simulink model "Prescan_Carsim_0118_cs"  (R2019b)
settings: Solver=ode5  StartTime=0.0  StopTime=inf  FixedStep=1/1000  RelTol=1e-3
PreLoadFcn:
  | mbxruntime.callbacks.PreLoadFcn(bdroot);
PostLoadFcn:
  | mbxruntime.callbacks.PostLoadFcn(bdroot);
InitFcn:
  | mbxruntime.callbacks.InitFcn(bdroot);
  | Initialization_Func;
  | 
  | % load the InputBus data.
  | load osqpcecInputBus.mat;
StartFcn:
  | mbxruntime.callbacks.StartFcn(bdroot);
  | current_sys=gcs;
  | speedblock=Simulink.findBlocks(current_sys,'Name','speed_kmh_Gain');
  | h1=add_exec_event_listener(speedblock,'PostOutputs',@SpeedVisulization);
  | outblock=Simulink.findBlocks(current_sys,'Name','trajectorycurveoutput_Gain');
  | CurveTrajectoryListenerHandle=add_exec_event_listener(outblock,'PostOutputs',@TrajectoryCurve_CallBack);
  | lanedatablock=Simulink.findBlocks(current_sys,'Name','LaneData_Gain');
  | CurveLaneListenerHandle=add_exec_event_listener(lanedatablock,'PostOutputs',@CurveLane_CallBack);
StopFcn:
  | mbxruntime.callbacks.StopFcn(bdroot);
model workspace: external: MAT-File .\Prescan_Carsim_0118_cs_hws.mat (data not in the file)
values from neighbouring files (symbols this model uses):
  g = 9.8    [Initialization_Func.m]
  InitialPlanningParameter = [0,0,1,0,2,2,2,40,60]'    [Initialization_Func.m]
  Kf = 20000    [Initialization_Func.m]
  Kr = 20000    [Initialization_Func.m]
  Lr = 1.644    [Initialization_Func.m]
  M = 1275    [Initialization_Func.m]
  nG = 24    [Initialization_Func.m]
  V = 60/3.6    (= 16.6666666667)    [Initialization_Func.m]
  VehicleBaseLength = Lf+Lr    (= 2.66)    [Initialization_Func.m]
undefined symbols (not defined in the file or in its folder): AAx, AAy, AAz, AVx, AVy, AVz, Ax, Ay, Az, canChannel, DiscIntNeverNeededParam, InitialDPMPDF_Comfort, InitialDPMPDF_Efficiency, InitialDPMPDF_Safety, InitialPDF_DEM, mbxruntime, NormalisedTrajectoryIndicator_Pool, Parameter_Indicator_LookUpTable, Prescan_Carsim_1230_cs_0658e9ca1334a8be, Prescan_Carsim_1230_cs_08c5eb9a1bd7376a, Prescan_Carsim_1230_cs_6cfd759b89b9fc85, Prescan_Carsim_1230_cs_9435cc1cceb5050d, Prescan_Carsim_1230_cs_ac716d34d49f74ab, Prescan_Carsim_1230_cs_be02757d7f212dd5, Rational_Coefficient_Learning, SteeringWheel, TrajectoryIndicatorRange, Vx, Vy, Vz, WheelL0, WheelL1, WheelR0, WheelR1
libraries: canmsglib x11, dsparch4 x6, canlib x3, PreScanSimulinkLibrary x3, Solver_SF x1, autolibshared x1
(part 6 of 8)

== matlab function Prescan_Carsim_0118_cs/BMW_X5_SUV_1/DEM updating and Preference Estimation/UpdateDEM/online DPM building preference estimation accordign to feedback/MATLAB Function ==
  data: FeedBack input; Real_Trajectory_Indicator input size=[1 3]; NormalisedTrajectoryIndicator_Pool input; ExpectedNext_NormalisedTrajectoryIndicator output; ExpectedNext_QueryID output; InitialPDF_DEM input; InitialDPMPDF_Safety input size=[1 2]; InitialDPMPDF_Comfort input size=[1 2]; InitialDPMPDF_Efficiency input size=[1 2]; TrajectoryIndicatorRange input; PostPDF_DEM output; PostDPMPDF_Safety output; Rational_Coefficient_Learning input; PostDPMPDF_Comfort output; PostDPMPDF_Effociency output
function [ExpectedNext_NormalisedTrajectoryIndicator,ExpectedNext_QueryID,PostPDF_DEM,PostDPMPDF_Safety,PostDPMPDF_Comfort,PostDPMPDF_Effociency]= fcn(FeedBack,Real_Trajectory_Indicator,NormalisedTrajectoryIndicator_Pool,InitialPDF_DEM,InitialDPMPDF_Safety,InitialDPMPDF_Comfort,InitialDPMPDF_Efficiency,TrajectoryIndicatorRange,Rational_Coefficient_Learning)
% Update the PDF_DEM and PDF_DPM according to the feedback, also select the
% trajectory indicators that would be shown to the driver for the following
% evaluation (compare)
% Query: The Trajectory Indicators array Num_Indicators*1;
% InitialPDF_DEM: a data array Num_WeightDEM*4, the first column is the
% pdf,and the 2-4 column are the weight of S-C-E
% InitialPDF_DPM: a 1*3 cell array, each cell is a data array like the
% PDF_DEM.

%============ Initialization ==============
persistent PriorPDF_DEM 
if isempty(PriorPDF_DEM)
    PriorPDF_DEM=InitialPDF_DEM;
end

persistent PriorDPMPDF_Safety
if isempty(PriorDPMPDF_Safety)
    PriorDPMPDF_Safety=InitialDPMPDF_Safety;
end

persistent PriorDPMPDF_Comfort
if isempty(PriorDPMPDF_Comfort)
    PriorDPMPDF_Comfort=InitialDPMPDF_Comfort;
end

persistent PriorDPMPDF_Efficiency
if isempty(PriorDPMPDF_Efficiency)
    PriorDPMPDF_Efficiency=InitialDPMPDF_Efficiency;
end

persistent Evaluated_NormalisedTrajectoryIndicator Step
if isempty(Evaluated_NormalisedTrajectoryIndicator)
    Step=1; 
    Evaluated_NormalisedTrajectoryIndicator=zeros(size(NormalisedTrajectoryIndicator_Pool,1),1);
    Real_NormalisedTrajectory_Indicator=DriverPerceptionModel(Real_Trajectory_Indicator,0,TrajectoryIndicatorRange);
    Diff_TrajectoryInd=NormalisedTrajectoryIndicator_Pool-repmat(Real_NormalisedTrajectory_Indicator,size(NormalisedTrajectoryIndicator_Pool,1),1);
    [~,Minimum_No]=min(sum(Diff_TrajectoryInd.^2,2));
    Evaluated_NormalisedTrajectoryIndicator(Step)=Minimum_No;      
end

persistent LastPreference_TrajectoryIndicator LastPreference_NormalisedTrajectoryIndicator
if isempty(LastPreference_TrajectoryIndicator)
    LastPreference_TrajectoryIndicator=Real_Trajectory_Indicator;
    LastPreference_NormalisedTrajectoryIndicator=DriverPerceptionModel(LastPreference_TrajectoryIndicator,0,TrajectoryIndicatorRange);
end
    
persistent PDF_WeightTable ID_PDFTable
if isempty(PDF_WeightTable)
    % Construct the WeightTable and the PDF_WeightTable by combining the
    % PDF_DEM and PDF_DPM
    Num_WeightDEM=size(PriorPDF_DEM,1);
    NumIndicator_DPM=[size(PriorDPMPDF_Safety,2)-1,size(PriorDPMPDF_Comfort,2)-1,size(PriorDPMPDF_Efficiency,2)-1];% zeros means only 1 indicator
    Num_WeightDPM=[size(PriorDPMPDF_Safety,1),size(PriorDPMPDF_Comfort,1),size(PriorDPMPDF_Efficiency,1)];
    PDF_WeightTable=zeros(prod(Num_WeightDPM)*Num_WeightDEM,sum(NumIndicator_DPM)+1);
    [X1,X2,X3,X4]=ndgrid((1:Num_WeightDPM(1))',(1:Num_WeightDPM(2))',(1:Num_WeightDPM(3))',(1: Num_WeightDEM)');
    ID_PDFTable=[X1(:),X2(:),X3(:),X4(:)];
    PDF_WeightTable(:,1)=PriorDPMPDF_Safety(X1(:),1).*PriorDPMPDF_Comfort(X2(:),1).*PriorDPMPDF_Efficiency(X3(:),1).*PriorPDF_DEM(X4(:),1);
    PDF_WeightTable(:,2:end)=[(PriorDPMPDF_Safety(X1(:),2:end).*PriorPDF_DEM(X4(:),2)),(PriorDPMPDF_Comfort(X2(:),2:end).*PriorPDF_DEM(X4(:),3)),...
        (PriorDPMPDF_Efficiency(X3(:),2:end).*PriorPDF_DEM(X4(:),4))];% The last three column is the weight of S-C-E 
end


% ============= Update the PDF_DEM and PDF_DPM =====================
% feedback:1 means prefer the first one, 2 means the second one, 3 means no preference,others menas no valid feedback
if FeedBack==1 || FeedBack==2 || FeedBack==3
    Step=Step+1;    
    % Calculate the current query position
    Real_NormalizedTrajectoryIndicator=DriverPerceptionModel(Real_Trajectory_Indicator,0,TrajectoryIndicatorRange);
    Diff_TrajectoryInd=NormalisedTrajectoryIndicator_Pool-repmat(Real_NormalizedTrajectoryIndicator,size(NormalisedTrajectoryIndicator_Pool,1),1);
    [~,Minimum_No]=min(sum(Diff_TrajectoryInd.^2,2));
    Evaluated_NormalisedTrajectoryIndicator(Step)=Minimum_No;
    
    if FeedBack==1 || FeedBack==2 
        Query=Real_NormalizedTrajectoryIndicator-LastPreference_NormalisedTrajectoryIndicator;
        % When Feedback is valid,update the PDF_DEM and PDF_DPM
        Compare_Result=FeedBack-1;% prefer the latter one? 1,means the second one
        LikeHood_Feedback=LikeHood_Func(PDF_WeightTable(:,2:end),Query,Compare_Result,Rational_Coefficient_Learning);
        Post_PDFWeight=PDF_WeightTable(:,1).*LikeHood_Feedback;
        % Update the PDF_DEM and PDF_DPM
        [PostPDF_DEM,~,PostDPMPDF_Safety,PostDPMPDF_Comfort,PostDPMPDF_Effociency,~]=UpdataPDF(Post_PDFWeight,PriorPDF_DEM,PriorDPMPDF_Safety,PriorDPMPDF_Comfort,PriorDPMPDF_Efficiency,ID_PDFTable); 
        %===
        PriorPDF_DEM=PostPDF_DEM;
        PriorDPMPDF_Safety=PostDPMPDF_Safety;
        PriorDPMPDF_Comfort=PostDPMPDF_Comfort;
        PriorDPMPDF_Efficiency=PostDPMPDF_Effociency;
        if FeedBack==2          
            LastPreference_TrajectoryIndicator=Real_Trajectory_Indicator;
            LastPreference_NormalisedTrajectoryIndicator=DriverPerceptionModel(LastPreference_TrajectoryIndicator,0,TrajectoryIndicatorRange);
        end        
    else
        % Do nothing,continue the next 
    end
    
end
PostPDF_DEM=PriorPDF_DEM;
PostDPMPDF_Safety=PriorDPMPDF_Safety;
PostDPMPDF_Comfort=PriorDPMPDF_Comfort;
PostDPMPDF_Effociency=PriorDPMPDF_Efficiency;

%======= Select the Next Trajectory Used to Commare for the next loop
%=================
% 1, Calculate the expected information difference for each possible query
% This one needs further modification
Available_ID=setdiff((1:size(NormalisedTrajectoryIndicator_Pool,1)),unique(Evaluated_NormalisedTrajectoryIndicator));
Alternative_Query=NormalisedTrajectoryIndicator_Pool(Available_ID,:)-repmat(LastPreference_NormalisedTrajectoryIndicator,length(Available_ID),1);
Max_QueryID=Select_ExpectedInformationVolume(PriorPDF_DEM,PriorDPMPDF_Safety,PriorDPMPDF_Comfort,PriorDPMPDF_Efficiency,PDF_WeightTable,ID_PDFTable,Alternative_Query,Rational_Coefficient_Learning);
ExpectedNext_QueryID=Available_ID(Max_QueryID);
ExpectedNext_NormalisedTrajectoryIndicator=NormalisedTrajectoryIndicator_Pool(ExpectedNext_QueryID,:);

end


%%
% Local Functions
function likehood= LikeHood_Func(WeightSet,Query,CompareResult,Rational_Coefficient_Learning)
% calculate each query's likolihood when the result was compare(0/1)
% WeightSet: should be column vecotrs Num_Weight*Num_Indicators,
% Query: should be a data array like Num_query*Num_Indicators
% 
% likehood is a data array like Num_Weight* Num_query, 
%     beta=5;% rationality coefficient 
coder.extrinsic('error');
    likehood=1./(1+exp(Rational_Coefficient_Learning*WeightSet*Query'));
    if CompareResult ==1
        return        
    elseif CompareResult==0
        likehood=1-likehood;
    else
        error ('False compare result!\n')
    end
end

function [PostPDF_DEM,SumPDFDEM_Post,PostPDFDPM_Safety,PostPDFDPM_Comfort,PostPDFDPM_Efficiency,SumDPMPDF_Post]=UpdataPDF(Post_PDFWeight,PriorPDF_DEM,PriorDPMPDF_Safety,PriorDPMPDF_Comfort,PriorDPMPDF_Efficiency,ID_PDFTable)
% Update the PDF_DEM
PostPDF_DEM=PriorPDF_DEM;
Num_Query=size(Post_PDFWeight,2);
if not(isempty(PriorPDF_DEM))
    Num_WeightDEM_temp=size(PriorPDF_DEM,1);
    % update the DEM
    PostPDF_DEMTemp=zeros(Num_WeightDEM_temp,Num_Query);
    for DEM_i=1:Num_WeightDEM_temp
        PostPDF_DEMTemp(DEM_i,:)=sum(Post_PDFWeight(ID_PDFTable(:,4)==DEM_i,:));
    end
    [PostPDF_DEMTemp,SumPDFDEM_Post]=PDF_NormFunc(PostPDF_DEMTemp,PriorPDF_DEM(:,2:end));
end
PostPDF_DEM(:,1)=PostPDF_DEMTemp;

% update the PDF_DPM
SumDPMPDF_Post=zeros(3,Num_Query);% 3*Num_Query
Num_WeightDPM=[size(PriorDPMPDF_Safety,1),size(PriorDPMPDF_Comfort,1),size(PriorDPMPDF_Efficiency,1)];

% Update the PDFDPM_Safety
PostPDFDPM_Safety=PriorDPMPDF_Safety;
PostPDF_DPMTemp=zeros(Num_WeightDPM(1),Num_Query);
for NumWeight_i=1:Num_WeightDPM(1)
    PostPDF_DPMTemp(NumWeight_i,:)=sum(Post_PDFWeight(ID_PDFTable(:,1)==NumWeight_i,:));
end
[PostDPMPDFWeight_Temp,SumPostPDFDPM_Temp]=PDF_NormFunc(PostPDF_DPMTemp,PriorDPMPDF_Safety(:,2:end));
PostPDFDPM_Safety(:,1)=PostDPMPDFWeight_Temp;
SumDPMPDF_Post(1,:)=SumPostPDFDPM_Temp;

% Update the PDFDPM_Comfort
PostPDFDPM_Comfort=PriorDPMPDF_Comfort;
PostPDF_DPMTemp=zeros(Num_WeightDPM(2),Num_Query);
for NumWeight_i=1:Num_WeightDPM(2)
    PostPDF_DPMTemp(NumWeight_i,:)=sum(Post_PDFWeight(ID_PDFTable(:,2)==NumWeight_i,:));
end
[PostDPMPDFWeight_Temp,SumPostPDFDPM_Temp]=PDF_NormFunc(PostPDF_DPMTemp,PriorDPMPDF_Comfort(:,2:end));
PostPDFDPM_Comfort(:,1)=PostDPMPDFWeight_Temp;
SumDPMPDF_Post(2,:)=SumPostPDFDPM_Temp;

% Update the PDFDPM_Efficiency
PostPDFDPM_Efficiency=PriorDPMPDF_Efficiency;
PostPDF_DPMTemp=zeros(Num_WeightDPM(3),Num_Query);
for NumWeight_i=1:Num_WeightDPM(3)
    PostPDF_DPMTemp(NumWeight_i,:)=sum(Post_PDFWeight(ID_PDFTable(:,3)==NumWeight_i,:));
end
[PostDPMPDFWeight_Temp,SumPostPDFDPM_Temp]=PDF_NormFunc(PostPDF_DPMTemp,PriorDPMPDF_Efficiency(:,2:end));
PostPDFDPM_Efficiency(:,1)=PostDPMPDFWeight_Temp;
SumDPMPDF_Post(3,:)=SumPostPDFDPM_Temp;
end

function [post_prob,sum_prob]=PDF_NormFunc(PDF,Weight_Set)
    % prob_distrib is a array of the post probability distribution. the row
    % number is the dicrete weight number,and the column number is the query/action.
    % each column is the post prob distribution of the query.
    % this function is to calculate the total prob in the considering
    % weight range to be 1
    % pdf_func: is a function handle.
   if size(PDF,1)==1
        post_prob=1;
        sum_prob=PDF;
    else
        uniqueweight=unique(Weight_Set(:,1));
        Interval_Weight=min(diff(uniqueweight));
        Ndim_ValidWeight=size(Weight_Set,2)-1;
        % considering the truth that the valid range of the independent variable
        if Ndim_ValidWeight==1
            sum_prob=sum(PDF(1:end-1))*Interval_Weight;
        else 
            pos_temp=sum(Weight_Set(:,1:Ndim_ValidWeight),2)<=1-Interval_Weight;
            sum_prob=sum(PDF(pos_temp,:))*Interval_Weight^Ndim_ValidWeight;
        end
        post_prob=PDF./repmat(sum_prob,size(PDF,1),1);
    end        
end

function max_queryID=Select_ExpectedInformationVolume(PriorPDF_DEM,PriorDPMPDF_Safety,PriorDPMPDF_Comfort,PriorDPMPDF_Efficiency,PDF_WeightTable,ID_PDFTable,Query_Pool,learning_rate_agent)
% calculate the expected difference between the prior and post probability
% density function for each query in the Query_Pool.
% PriorPDF_DEM: initial prob distribution of the DEM(S-C-E),Num_Weight_DEM*1;
% DEM_WeightSet : date array like Ndim*Num_discrete_theta
% Query_pool:data array like Ndim*Num_query
Num_Query=size(Query_Pool,1);
DEM_WeightSet=PriorPDF_DEM(:,2:end);
Num_WeightDEM=size(PriorPDF_DEM,1);

PDF_WeightTable(:,1)=PriorDPMPDF_Safety(ID_PDFTable(:,1),1).*PriorDPMPDF_Comfort(ID_PDFTable(:,2),1).*PriorDPMPDF_Efficiency(ID_PDFTable(:,3),1).*PriorPDF_DEM(ID_PDFTable(:,4),1);
LikeHood_1_WeightByQuery=LikeHood_Func(PDF_WeightTable(:,2:end),Query_Pool,1,learning_rate_agent);
Post_PDF=repmat(PDF_WeightTable(:,1),1,Num_Query).*LikeHood_1_WeightByQuery;

% the expected information difference of DEM
PostPDF_DEM=zeros(Num_WeightDEM,Num_Query);
for DEM_i=1:Num_WeightDEM
    PostPDF_DEM(DEM_i,:)=sum(Post_PDF(ID_PDFTable(:,4)==DEM_i,:),1);
end

[Post_PDFNorm,sum_post]=PDF_NormFunc(PostPDF_DEM,DEM_WeightSet);


Prob_Difference=abs(repmat(PriorPDF_DEM(:,1),1,Num_Query)-Post_PDFNorm);
[~,Sum_Prob_Difference]=PDF_NormFunc(Prob_Difference,DEM_WeightSet);
Expected_Information=Sum_Prob_Difference.*sum_post;
[~,max_queryID]=max(Expected_Information);
end

function TrajectoryIndicator_Perceived=DriverPerceptionModel(TrajectoryIndicator,Flag,TrajectoryIndicatorRange)
% Flag: 0 means to transform the real trajectory indicator into Normalized
% Trajectory Indicators, vice versa, 1 means transform the normalized into
% real trajectory indicators

% RightLateralOffset,LateralAcceleration,Time
% Minimum_TrajectoryIndicator=[0,0.4,14];
% Maximum_TrajectoryIndicator=[0.5,3.4,18];
Minimum_TrajectoryIndicator=TrajectoryIndicatorRange(1,:);
Maximum_TrajectoryIndicator=TrajectoryIndicatorRange(2,:);

if Flag==1
    Normalized_TrajectoryIndicator=TrajectoryIndicator;
    TrajectoryIndicator_Perceived=Minimum_TrajectoryIndicator+(Maximum_TrajectoryIndicator-Minimum_TrajectoryIndicator).*Normalized_TrajectoryIndicator;
    % This is special for the LateralOffset_Right
    TrajectoryIndicator_Perceived(1)=-1*TrajectoryIndicator_Perceived(1);
elseif Flag==0
    %==== These are refered to the DriverPerceptionBase.m
    % JND-just noticeable difference
    %Can You Feel The Difference? The Just Noticeable Difference of
    %Longitudinal Acceleration, http://sage.cnpereading.com/paragraph/article/?doi=10.1177/1541931213571271
    JND_Acceleration=0.1;
    % Lateral Offset, Assume Left and Right be tha same,and to be 0.1m;
    JND_LateralOffset=0.1;%
    % Time, Or May be the Average Time would be More Significant
    JND_Time=2;
    
    GridIndicator=zeros(3,size(Minimum_TrajectoryIndicator,2));
    GridIndicator(1,:)=(Minimum_TrajectoryIndicator+eps)./[JND_LateralOffset,JND_Acceleration,JND_Time];
    GridIndicator(2,:)=(Maximum_TrajectoryIndicator+eps)./[JND_LateralOffset,JND_Acceleration,JND_Time];
    GridIndicator(3,:)=(abs(TrajectoryIndicator)+eps)./[JND_LateralOffset,JND_Acceleration,JND_Time];
    
    TrajectoryIndicator_Perceived=(GridIndicator(3,:)-GridIndicator(1,:))./(GridIndicator(2,:)-GridIndicator(1,:));
    TrajectoryIndicator_Perceived(TrajectoryIndicator_Perceived<0)=0;
    TrajectoryIndicator_Perceived(TrajectoryIndicator_Perceived>1)=1;
end
end

== matlab function Prescan_Carsim_0118_cs/BMW_X5_SUV_1/trajectory planning/A substitution for the above trajectory planning subsystem/Trajectory Planning When Not Curve ==
  data: RoadLane_Plan input size=[1000 4]; Path_Plan output size=[1000 2]; Speed_Planned_kmh output size=[1000 1]; MaxSpeed input; PlanPathDataLength_Straight output size=1
function [Path_Plan,Speed_Planned_kmh,PlanPathDataLength_Straight]= fcn(RoadLane_Plan,MaxSpeed)

%Road Lane
LeftLane_Plan=RoadLane_Plan(:,1:2);
RightLane_Plan=RoadLane_Plan(:,3:4);
Num_LanePlan=size(RightLane_Plan,1);
Path_PlanTemp=zeros(1000,2);

X_LeftToRight=RightLane_Plan(:,1)-LeftLane_Plan(:,1);%const 2
Y_LeftToRight=RightLane_Plan(:,2)-LeftLane_Plan(:,2);

alpha=0.5*ones(Num_LanePlan,1); % Lane centering
Path_PlanTemp(1:Num_LanePlan,1) = LeftLane_Plan(:,1) + X_LeftToRight.* alpha;
Path_PlanTemp(1:Num_LanePlan,2)= LeftLane_Plan(:,2) + Y_LeftToRight.* alpha;
% Path_Plan=Path_PlanTemp(1:Num_LanePlan,:);
Path_Plan=Path_PlanTemp;
PlanPathDataLength_Straight=Num_LanePlan;
% Speed_Planned_kmh=Constant_Speed*ones(Num_LanePlan,1);
Speed_Planned_kmh=MaxSpeed*ones(1000,1);
%Trajectory=[Path_Plan,Speed_Planned_kmh];

% smooth or interplate the trajecotry 

end

== matlab function Prescan_Carsim_0118_cs/BMW_X5_SUV_1/trajectory planning/Specific Curve Trajectory Planning/Convert Curve Path To Local (under vehicle) ==
  data: PathPlan_Global input size=[1000 2]; VehicleState_Global input; PathPlan_Local output size=[1000 2]
function PathPlan_Local =fcn(PathPlan_Global,VehicleState_Global)
% Convert the global path to local(different with the local under beginning
%  position.
X_TargetPath=PathPlan_Global(:,1);
Y_TargetPath=PathPlan_Global(:,2);
HeadingAngle_rad=VehicleState_Global(3);
PathPlan_Local =([X_TargetPath - VehicleState_Global(1),Y_TargetPath-VehicleState_Global(2)])*[cos(HeadingAngle_rad) sin(HeadingAngle_rad); -sin(HeadingAngle_rad) cos(HeadingAngle_rad)]';  % 将原始参考路径旋转平移至车辆坐标系下
end

== matlab function Prescan_Carsim_0118_cs/BMW_X5_SUV_1/trajectory planning/Subsystem/Determination of Curve Road No/Determine Curve No According the vehicle position ==
  data: VehicleState_Global input; Curve_No output
function Curve_No = fcn(VehicleState_Global)
X_Global=VehicleState_Global(1);
Y_Global=VehicleState_Global(2);
% These coordinates was from the scenery in pex GUI
if X_Global>=20 && Y_Global>=-182.7
    %Y_Global>=150 && Y_Global<=300.6
    % This is not very accurate
    Curve_No=1;
elseif X_Global>=20 && Y_Global<=-272.7
    %Y_Global>=400.6 && Y_Global<=554.247
    Curve_No=2;
elseif X_Global<=-70 && Y_Global<=-272.7
    Curve_No=3;
elseif X_Global<=-70 && Y_Global>=-182.7
    Curve_No=4;    
else
    Curve_No=0;
end

== matlab function Prescan_Carsim_0118_cs/BMW_X5_SUV_1/trajectory tracking Information/Preview Information Calculation 2 ==
  data: TargetPath_Local input size=[1000 2]; Offset_Preview output; HeadError_rad output; Curvature_Vehicle output; TargetSpeed_Plan input size=[1000 1]; TrackingError output; PreviewDistance output; TargetSpeed_Current output
function [Offset_Preview,HeadError_rad,Curvature_Vehicle,TrackingError,PreviewDistance,TargetSpeed_Current] = fcn(TargetPath_Local,TargetSpeed_Plan)
% calculate the preview information used in the SMC controller

Path_UnderVehicleCoordinates=TargetPath_Local;
% Target speed for current vehicle position
% Pick up the speed points close to the vehicle, within range(-15,15)
Speed_CloseToVehicle= TargetSpeed_Plan(Path_UnderVehicleCoordinates(:,1)<=15 ...
    & Path_UnderVehicleCoordinates(:,1)>=-15,:);
ID_CloseToVehicle= Path_UnderVehicleCoordinates(Path_UnderVehicleCoordinates(:,1)<=15 ...
    & Path_UnderVehicleCoordinates(:,1)>=-15,:);
% % spline
TargetSpeed_Current = spline(ID_CloseToVehicle(:,1), Speed_CloseToVehicle, 0);% current speed
PreviewDistance=0.072*TargetSpeed_Current+5;% used to calculate the preview error

%Pick up the path points close to the preview point
Path_CloseToPreview= Path_UnderVehicleCoordinates(Path_UnderVehicleCoordinates(:,1)<= 2*PreviewDistance & Path_UnderVehicleCoordinates(:,1)>=0,:);
%spline
Interval_spline = 0.01;
Xeq = (0 : Interval_spline : Path_CloseToPreview(end,1))';
Yeq = spline(Path_CloseToPreview(:,1), Path_CloseToPreview(:,2), Xeq);
PathCloseToPreview_spline=[Xeq,Yeq];
%Calculate the lateral offset of the preview point，
%Positive if the preview point is on the left of the target path,vice versa
Preview_Point=[PreviewDistance,0];
[Offset_Preview,~,~]=DistanceCurvature_Calculate(PathCloseToPreview_spline,Preview_Point,0,0);


%Calculate the curvature of the target path that close to the vehicle,
% Positive if the target path curve is left curve, vice versa
%Pick up the path points close to the vehicle
Path_CloseToVehicle= Path_UnderVehicleCoordinates(Path_UnderVehicleCoordinates(:,1)<=2*PreviewDistance ...
    & Path_UnderVehicleCoordinates(:,1)>=-2*PreviewDistance,:);
%spline
Xeq = (-2*PreviewDistance : Interval_spline : Path_CloseToVehicle(end,1))';
Yeq = spline(Path_CloseToVehicle(:,1), Path_CloseToVehicle(:,2), Xeq);
PathCloseToVehicle_spline=[Xeq,Yeq];
[TrackingError,Curvature_Vehicle,HeadError_rad]=DistanceCurvature_Calculate(PathCloseToVehicle_spline,[0,0],1,1);

% Visulization
% Plot_Preview_Local(TargetPath_Local,Distance_Preview)
end

%%
%local functions
function [DistanceToPoint,Curvature,HeadError]=DistanceCurvature_Calculate(Path,Target_Point,Curvature_Cal,HeadError_Cal)
% #codegen
coder.extrinsic('warning');
[~, Id_min]=min((Target_Point(1)-Path(:,1)).^2+(Target_Point(2)-Path(:,2)).^2);
if (Id_min < size(Path,1)-10)
    vec_Path = [Path(Id_min+10,:),0]-[Path(Id_min,:),0];
    vec_TargetToPath = [Target_Point,0]-[Path(Id_min,:),0];
else
    vec_Path = [Path(Id_min,:),0]-[Path(Id_min-10,:),0];
    vec_TargetToPath = [Target_Point,0]-[Path(Id_min-10,:),0];
end
Cross_VecPretoPath_VecPath=cross(vec_Path,vec_TargetToPath);
DistanceToPoint=Cross_VecPretoPath_VecPath(:,3)./sqrt(sum(vec_Path.*vec_Path));
% DistanceToPoint=sqrt(DisSquare_PreToPath);
Sin_Angle=abs(DistanceToPoint)/sqrt(sum(vec_TargetToPath.*vec_TargetToPath));
if Sin_Angle<sin(deg2rad(85))
    warning('The calcuated lateral distance of preview point to path is not very accurate!');
end

HeadError=0;
if HeadError_Cal==1
   Vec_Vehicle=[1,0,0];
%    if (Id_min < size(Path,1))
%       vec_Path2=[Path(Id_min+1,:),0]-[Path(Id_min,:),0];
%    else
%       vec_Path2 = [Path(Id_min,:),0]-[Path(Id_min-1,:),0];
%    end
   Cross_VehicleToPath=cross(vec_Path,Vec_Vehicle);
   Sin_Angle=Cross_VehicleToPath(3)/sqrt(sum(vec_Path.*vec_Path));
   HeadError=asin(Sin_Angle);   
end

Curvature=0;
if Curvature_Cal==1
    Radius_ChooseDataForCur=300;% about 3m for interval 0.01.
    if Id_min<=size(Path,1)-Radius_ChooseDataForCur && Id_min>=Radius_ChooseDataForCur
        Id_Lower=Id_min-Radius_ChooseDataForCur+1;
        Id_Upper=Id_min+Radius_ChooseDataForCur;
    elseif Id_min>size(Path,1)-Radius_ChooseDataForCur
        Id_Upper=size(Path,1);
        Id_Lower=max(size(Path,1)-2*Radius_ChooseDataForCur,1);        
    elseif Id_min<Radius_ChooseDataForCur
        Id_Lower=1;
        Id_Upper=min(2*Radius_ChooseDataForCur,size(Path,1));
    else
        warning('The curvature calculation is something wrong!');
        Curvature=0;
        return
    end
    %{
    % Method 1
    Path_cur=Path(Id_Lower:Id_Upper,:);
    A=[Path_cur,ones(size(Path_cur,1),1)];
    if rank(A) ~= size(A,2)
        Curvature= 0;
    else
        B=-1*sum(Path_cur.*Path_cur,2);
        coef=A\B;%圆一般方程式的的系数DEF
        Curvature=2/sqrt(coef(1)^2+coef(2)^2-4*coef(3));
        if Curvature<1/1000
            Curvature=0;
        end
    end
    %}
    % Method 2 another method with 3 points, but maybe unstable
    vec1 = [Path(Id_min,:)-Path(Id_Lower,:),0];
    vec2 = [Path(Id_Upper,:)-Path(Id_min,:),0];
    z1 =Path(Id_min,:)*Path(Id_min,:)'-Path(Id_Lower,:)*Path(Id_Lower,:)';
    z2 =Path(Id_Upper,:)*Path(Id_Upper,:)'-Path(Id_Lower,:)*Path(Id_Lower,:)';
    z3 =Path(Id_Upper,:)*Path(Id_Upper,:)'-Path(Id_min,:)*Path(Id_min,:)'; 
    direction  = cross(vec1,vec2);
    sin_theta=abs(direction(3))/(sqrt(vec1*vec1')*sqrt(vec2*vec2'));
    curvature_estimate=asin(sin_theta)/(sqrt(vec2*vec2'));% the theta/length
    if curvature_estimate>1/1000  
        % the curvatrue_estimate is larger than 1/1000(Radius is smaller than 1000),the old is the direction(3) is
        % larger than 1e-9;
        A = [Path(Id_min,:)-Path(Id_Lower,:); Path(Id_Upper,:)-Path(Id_Lower,:); Path(Id_Upper,:)-Path(Id_min,:)];
        B = 0.5*[z1;  z2;  z3];
        P0 = (A'*A)\A'*B;
        R1 =sqrt((P0'-Path(Id_Lower,:))*(P0'-Path(Id_Lower,:))');
        R2 =sqrt((P0'-Path(Id_min,:))*(P0'-Path(Id_min,:))');
        R3 =sqrt((P0'-Path(Id_Upper,:))*(P0'-Path(Id_Upper,:))');
        R = (R1 + R2 + R3)/3;
        Curvature = 1/R*sign(direction(3));
    else
        Curvature = 0;
    end
    %}
end
end

== matlab function Prescan_Carsim_0118_cs/BMW_X5_SUV_1/Tracking Control & vehicle dynamics/Lane Keeping Assistance/Path Tracking - SMC controller ==
  data: c1 input; c2 input; delta input; kapa input; PreviewError input; PreviewError_dot input; HeadingError input; HeadingError_dot input; Curvature input; SteerAngle output; PreviewDistance input; v input
function SteerAngle = fcn( c1, c2, delta, kapa, PreviewError, PreviewError_dot, HeadingError, HeadingError_dot, Curvature,PreviewDistance,v)
% 滑膜控制参数定义
%先定义车辆本身的参数
g=9.8;%重力加速度m/s^2
M=1396; %车辆的质量kg
I=2204; %车辆的横摆转动惯量kg·m2
Kf=50192; %前轮的侧偏刚度Nm/rad
Kr=50192; %后轮的侧偏刚度Nm/rad
Lf=1.01; %车辆质心到前轴的距离m
Lr=1.59; %车辆质心到后轴的距离m
%待调参数： 预瞄时长t_pre, 滑膜面参数 c1, c2, 趋近率参数delta, kapa
%输入参数； 预瞄偏差ep,  参考航向角phi_d, 本车航向角 phi, 道路曲率 qulv  航向角偏差影响系数 phir_k0 phir_k1
phir_k0 = 0.85;
phir_k1 = 0.85;
L = PreviewDistance; %车辆预瞄距离设定
smc_a12 = -(1+(Lf*Kf-Lr*Kr)/(M*v^2));
smc_a34 = (Kf+Kr)/M+L*(Kf*Lf-Kr*Lr)/I;
smc_a35 = L*(Kf+Kr)/(M*v)-(Kf*Lf-Kr*Lr)/(M*v)+L^2*(Kf*Lf-Kr*Lr)/(I*v)-L*(Kf*Lf^2+Kr*Lr^2)/(I*v);
smc_a36 = (Kf+Kr)/(M*v)+L*(Kf*Lf-Kr*Lr)/(I*v);
smc_b32 = (L*Kf*Lf)/I+Kf/M;
smc_d32 = -(v+(Kf*Lf-Kr*Lr)/(M*v)-L*smc_a12);
ep_cum = 0;
s1 = PreviewError_dot + c1 * PreviewError + c2 * ep_cum;
f1 = smc_a34 * HeadingError*phir_k0 + smc_a35 * HeadingError_dot*phir_k1 + c2 * PreviewError + (smc_a36+c1)*PreviewError_dot;
t1 = (1-exp(-10*s1))./(1+exp(-10*s1));
smc_ur = -1/smc_b32*(delta*t1 + kapa*s1 + f1 + smc_d32*v*Curvature);
k3 = smc_a34/smc_b32;
smc_uf = (M*v^2*Curvature)/(2*(Lf+Lr))*(Lr/Kf-Lf/Kr+Lf/Kr*k3)+Curvature*((Lf+Lr)-Lr*k3);
smc_u = smc_uf*0.03*(0) + smc_ur;
SteerAngle = smc_u;

== matlab function Prescan_Carsim_0118_cs/BMW_X5_SUV_1/trajectory planning/A substitution for the above trajectory planning subsystem/Convert Curve Path To Local (under vehicle) ==
  data: PathPlan_Global input size=[1000 2]; VehicleState_CurvePlanningBegining input size=[1 3]; VehicleState_Global input; PathPlan_Local output size=[1000 2]
function PathPlan_Local =fcn(PathPlan_Global,VehicleState_CurvePlanningBegining,VehicleState_Global)
% #codegen
% Convert the local path to global path
HeadingAngle_Beginning_rad=deg2rad(VehicleState_CurvePlanningBegining(3));
Rotation_Beginning=[cos(HeadingAngle_Beginning_rad),-sin(HeadingAngle_Beginning_rad); sin(HeadingAngle_Beginning_rad),cos(HeadingAngle_Beginning_rad)];
PathPlan_Beginning_temp=PathPlan_Global(:,1:2)*Rotation_Beginning';
PathPlan_Beginning=[PathPlan_Beginning_temp(:,1)+VehicleState_CurvePlanningBegining(1),...
    PathPlan_Beginning_temp(:,2)+VehicleState_CurvePlanningBegining(2)];

% Convert the global path to local(different with the local under beginning
%  position.
X_TargetPath=PathPlan_Beginning(:,1);
Y_TargetPath=PathPlan_Beginning(:,2);
HeadingAngle_rad=deg2rad(VehicleState_Global(3));
PathPlan_Local =([X_TargetPath - VehicleState_Global(1),Y_TargetPath-VehicleState_Global(2)])*[cos(HeadingAngle_rad) sin(HeadingAngle_rad); -sin(HeadingAngle_rad) cos(HeadingAngle_rad)]';  % 将原始参考路径旋转平移至车辆坐标系下
end

== matlab function Prescan_Carsim_0118_cs/BMW_X5_SUV_1/trajectory planning/A substitution for the above trajectory planning subsystem/MATLAB Function ==
  data: PathPlan_FixedSize input; TargetPath_VariableSize output size=[1000 2]; PlanSpeed_FixedSize input; TargetSpeed_VariableSize output size=[1000 1]; DataLength_Plan input
function [TargetPath_VariableSize,TargetSpeed_VariableSize]  = fcn(PathPlan_FixedSize,PlanSpeed_FixedSize,DataLength_Plan)
TargetPath_VariableSize=PathPlan_FixedSize(1:DataLength_Plan,:);
TargetSpeed_VariableSize = PlanSpeed_FixedSize(1:DataLength_Plan,:);
end

== matlab function Prescan_Carsim_0118_cs/BMW_X5_SUV_1/DriverFeedBack/driver evaluation model/Simulated Driver ==
  data: TrajectoryIndicator input size=[1 3]; Preference_DEM input; Compare_Result output; FeedBack_Count output; PreferenceDPM_Safety input; PreferenceDPM_Comfort input; PreferenceDPM_Efficiency input; Rational_coefficient input; Driver_Type input; mis_answered_ind output
function [Compare_Result,FeedBack_Count,mis_answered_ind]=Driver_Compare(TrajectoryIndicator,Preference_DEM,PreferenceDPM_Safety,PreferenceDPM_Comfort,PreferenceDPM_Efficiency,Rational_coefficient,Driver_Type)
%#codegen
% preference should be a column vector Ndim*1;
% query should be a data array Ndim*Num_query
% varargin- 'driver type', the list value include{'complete_rational','probability_rational','bound_rational'}
%  'bound_rational': when the probability of prefered is larger than a
%  upper_bound, the answer is 1; or when the probability of prefered is
%  less than a lower bound, the answer is 0; else the probability within
%  [lower_bound, upper_bound], the driver answers according to the
%  probability.
% Preference_DEM:3*1
coder.extrinsic('error');

persistent FeedBack_trigger
if isempty(FeedBack_trigger)
    FeedBack_trigger=0;
end

persistent LastPreference_TrajectoryIndicator_Driver
if isempty(LastPreference_TrajectoryIndicator_Driver)
    LastPreference_TrajectoryIndicator_Driver=TrajectoryIndicator;
end

persistent InitialFlag
if isempty(InitialFlag)
    InitialFlag=1;
end

mis_answered_ind=0;
if InitialFlag==1
    Compare_Result=-1;
    InitialFlag=0;
else    
    Query=TrajectoryIndicator-LastPreference_TrajectoryIndicator_Driver;
    Num_query=size(Query,1);
    Compare_Result=zeros(Num_query,1);
    Preference=[Preference_DEM(1)*PreferenceDPM_Safety(1,:),Preference_DEM(2)*PreferenceDPM_Comfort(1,:),Preference_DEM(3)*PreferenceDPM_Efficiency(1,:)];
    prob_1=LikeHood_Func(Preference,Query,1,Rational_coefficient);    
    if Driver_Type==1
        %"complete_rational"
        Compare_Result(prob_1>0.5)=1;
    elseif Driver_Type==2
        %"probability_rational"
        r1=rand(1,Num_query);
        Compare_Result(prob_1>r1)=1;
        False_negative=prob_1>0.5 & Compare_Result==0;
        False_positive=prob_1<0.5 & Compare_Result==1;
        mis_answered_ind=double(False_negative | False_positive);
    else 
        % "bound_rational"
        upper_bound=0.6;
        lower_bound=0.4;
        Compare_Result(prob_1>upper_bound)=1;
        prob_ind=prob_1>lower_bound & prob_1<= upper_bound;
        Compare_Result(prob_ind)=2;
        False_negative=prob_1>0.5 & Compare_Result==0;
        False_positive=prob_1<0.5 & Compare_Result==1;
        mis_answered_ind=double(False_negative | False_positive);         
    end
    if isequal(FeedBack_trigger,0)
        FeedBack_trigger=1;
    else
        FeedBack_trigger=0;
    end
end

FeedBack_Count=FeedBack_trigger;
Compare_Result=Compare_Result+1;
if Compare_Result==2
    LastPreference_TrajectoryIndicator_Driver=TrajectoryIndicator;
end
end

== matlab function Prescan_Carsim_0118_cs/BMW_X5_SUV_1/trajectory planning/Out of Specific Curve Planning/Trajectory Planning When Not Curve ==
  data: RoadLane_Plan input size=[1000 4]; Path_Plan output size=[1000 2]; Speed_Planned_kmh output size=[1000 1]; MaxSpeed input; PlanPathDataLength_Straight output size=1
function [Path_Plan,Speed_Planned_kmh,PlanPathDataLength_Straight]= fcn(RoadLane_Plan,MaxSpeed)

%Road Lane
LeftLane_Plan=RoadLane_Plan(:,1:2);
RightLane_Plan=RoadLane_Plan(:,3:4);
Num_LanePlan=size(RightLane_Plan,1);
Path_PlanTemp=zeros(1000,2);

X_LeftToRight=RightLane_Plan(:,1)-LeftLane_Plan(:,1);%const 2
Y_LeftToRight=RightLane_Plan(:,2)-LeftLane_Plan(:,2);

alpha=0.5*ones(Num_LanePlan,1); % Lane centering
Path_PlanTemp(1:Num_LanePlan,1) = LeftLane_Plan(:,1) + X_LeftToRight.* alpha;
Path_PlanTemp(1:Num_LanePlan,2)= LeftLane_Plan(:,2) + Y_LeftToRight.* alpha;
% Path_Plan=Path_PlanTemp(1:Num_LanePlan,:);
Path_Plan=Path_PlanTemp;
PlanPathDataLength_Straight=Num_LanePlan;
% Speed_Planned_kmh=Constant_Speed*ones(Num_LanePlan,1);
Speed_Planned_kmh=MaxSpeed*ones(1000,1);
%Trajectory=[Path_Plan,Speed_Planned_kmh];

% smooth or interplate the trajecotry 

end

== matlab function Prescan_Carsim_0118_cs/BMW_X5_SUV_1/DEM updating and Preference Estimation/UpdateDEM/Trajectory Planning Parameter Management1/Determine planning parameter according to the expected TrajectoryIndicators_LookUpTable ==
  data: IntialTrajectoryPlanningParameter input; PlanningParameter output; unused input; ExpectedNext_QueryID input; Parameter_IndicatorLookUpTable input
function PlanningParameter = fcn(IntialTrajectoryPlanningParameter,~,ExpectedNext_QueryID,Parameter_IndicatorLookUpTable)

persistent Parameter_Indicator_LookUpTable
if isempty(Parameter_Indicator_LookUpTable)
    Parameter_Indicator_LookUpTable=Parameter_IndicatorLookUpTable;
end
% if it is the first tiem
persistent Flag
if isempty(Flag)
    Flag=0;
end

persistent Intial_PlanningParameter
if isempty(Intial_PlanningParameter)
    Intial_PlanningParameter=IntialTrajectoryPlanningParameter;
end

if Flag==0
    PlanningParameter=Intial_PlanningParameter;
else
    PlanningParameter=Parameter_Indicator_LookUpTable(ExpectedNext_QueryID,1:9)';
end
Flag=1;
end

== matlab function Prescan_Carsim_0118_cs/BMW_X5_SUV_1/DEM updating and Preference Estimation/UpdateDEM/Online DEM updating/UPdate DEM ==
  data: FeedBack input; Query input size=[1 3]; PriorPDF_DEM input; PriorDPMPDF_Safety input size=[1 2]; PriorDPMPDF_Comfort input size=[1 2]; PriorDPMPDF_Efficiency input size=[1 2]; PostPDF_DEM output; PostDPMPDF_Safety output; Rational_Coefficient_Learning input; PostDPMPDF_Comfort output; PostDPMPDF_Effociency output
function [PostPDF_DEM,PostDPMPDF_Safety,PostDPMPDF_Comfort,PostDPMPDF_Effociency]= fcn(FeedBack,Query,PriorPDF_DEM,PriorDPMPDF_Safety,PriorDPMPDF_Comfort,PriorDPMPDF_Efficiency,Rational_Coefficient_Learning)
% Update the PDF_DEM and PDF_DPM according to the feedback, also select the
% trajectory indicators that would be shown to the driver for the following
% evaluation (compare)
% Query: The Trajectory Indicators array Num_Indicators*1;
% InitialPDF_DEM: a data array Num_WeightDEM*4, the first column is the
% pdf,and the 2-4 column are the weight of S-C-E
% InitialPDF_DPM: a 1*3 cell array, each cell is a data array like the
% PDF_DEM.

%============ Initialization ==============  

persistent Prior_DEM 
if isempty(Prior_DEM)
    Prior_DEM=PriorPDF_DEM;
end

persistent PriorDPM_Safety
if isempty(PriorDPM_Safety)
    PriorDPM_Safety=PriorDPMPDF_Safety;
end

persistent PriorDPM_Comfort
if isempty(PriorDPM_Comfort)
    PriorDPM_Comfort=PriorDPMPDF_Comfort;
end

persistent PriorDPM_Efficiency
if isempty(PriorDPM_Efficiency)
    PriorDPM_Efficiency=PriorDPMPDF_Efficiency;
end

persistent PDF_WeightTable ID_PDFTable
if isempty(PDF_WeightTable)
    % Construct the WeightTable and the PDF_WeightTable by combining the
    % PDF_DEM and PDF_DPM
    Num_WeightDEM=size(PriorPDF_DEM,1);
    NumIndicator_DPM=[size(PriorDPMPDF_Safety,2)-1,size(PriorDPMPDF_Comfort,2)-1,size(PriorDPMPDF_Efficiency,2)-1];% zeros means only 1 indicator
    Num_WeightDPM=[size(PriorDPMPDF_Safety,1),size(PriorDPMPDF_Comfort,1),size(PriorDPMPDF_Efficiency,1)];
    PDF_WeightTable=zeros(prod(Num_WeightDPM)*Num_WeightDEM,sum(NumIndicator_DPM)+1);
    [X1,X2,X3,X4]=ndgrid((1:Num_WeightDPM(1))',(1:Num_WeightDPM(2))',(1:Num_WeightDPM(3))',(1: Num_WeightDEM)');
    ID_PDFTable=[X1(:),X2(:),X3(:),X4(:)];
%   PDF_WeightTable(:,1)=PriorDPMPDF_Safety(X1(:),1).*PriorDPMPDF_Comfort(X2(:),1).*PriorDPMPDF_Efficiency(X3(:),1).*PriorPDF_DEM(X4(:),1);
    PDF_WeightTable(:,2:end)=[(PriorDPMPDF_Safety(X1(:),2:end).*PriorPDF_DEM(X4(:),2)),(PriorDPMPDF_Comfort(X2(:),2:end).*PriorPDF_DEM(X4(:),3)),...
        (PriorDPMPDF_Efficiency(X3(:),2:end).*PriorPDF_DEM(X4(:),4))];% The last three column is the weight of S-C-E 
end
PDF_WeightTable(:,1)=PriorDPMPDF_Safety(ID_PDFTable(:,1),1).*PriorDPMPDF_Comfort(ID_PDFTable(:,2),1).*PriorDPMPDF_Efficiency(ID_PDFTable(:,3),1).*PriorPDF_DEM(ID_PDFTable(:,4),1);

% ============= Update the PDF_DEM and PDF_DPM =====================
% feedback:1 means prefer the first one, 2 means the second one, 3 means no preference,others menas no valid feedback    
if FeedBack==1 || FeedBack==2 
    % When Feedback is valid,update the PDF_DEM and PDF_DPM
    Compare_Result=FeedBack-1;% prefer the latter one? 1,means the second one
    LikeHood_Feedback=LikeHood_Func(PDF_WeightTable(:,2:end),Query,Compare_Result,Rational_Coefficient_Learning);
    Post_PDFWeight=PDF_WeightTable(:,1).*LikeHood_Feedback;
    % Update the PDF_DEM and PDF_DPM
    [PostPDF_DEMtemp,~,PostDPMPDF_Safetytemp,PostDPMPDF_Comforttemp,PostDPMPDF_Effociencytemp,~]=UpdataPDF(Post_PDFWeight,PriorPDF_DEM,PriorDPMPDF_Safety,PriorDPMPDF_Comfort,PriorDPMPDF_Efficiency,ID_PDFTable); 
    Prior_DEM=PostPDF_DEMtemp;
    PriorDPM_Safety=PostDPMPDF_Safetytemp;
    PriorDPM_Comfort=PostDPMPDF_Comforttemp;
    PriorDPM_Efficiency=PostDPMPDF_Effociencytemp;
else
    % if no preference,(the two have no obvious difference)==============
    % Do nothing,continue the next 
end    

PostPDF_DEM=Prior_DEM;
PostDPMPDF_Safety=PriorDPM_Safety;
PostDPMPDF_Comfort=PriorDPM_Comfort;
PostDPMPDF_Effociency=PriorDPM_Efficiency;

end


%%
% Local Functions
function likehood= LikeHood_Func(WeightSet,Query,CompareResult,Rational_Coefficient_Learning)
% calculate each query's likolihood when the result was compare(0/1)
% WeightSet: should be column vecotrs Num_Weight*Num_Indicators,
% Query: should be a data array like Num_query*Num_Indicators
% 
% likehood is a data array like Num_Weight* Num_query, 
%     beta=5;% rationality coefficient 
coder.extrinsic('error');
    likehood=1./(1+exp(Rational_Coefficient_Learning*WeightSet*Query'));
    if CompareResult ==1
        return        
    elseif CompareResult==0
        likehood=1-likehood;
    else
        error ('False compare result!\n')
    end
end

function [PostPDF_DEM,SumPDFDEM_Post,PostPDFDPM_Safety,PostPDFDPM_Comfort,PostPDFDPM_Efficiency,SumDPMPDF_Post]=UpdataPDF(Post_PDFWeight,PriorPDF_DEM,PriorDPMPDF_Safety,PriorDPMPDF_Comfort,PriorDPMPDF_Efficiency,ID_PDFTable)
% Update the PDF_DEM
PostPDF_DEM=PriorPDF_DEM;
Num_Query=size(Post_PDFWeight,2);
if not(isempty(PriorPDF_DEM))
    Num_WeightDEM_temp=size(PriorPDF_DEM,1);
    % update the DEM
    PostPDF_DEMTemp=zeros(Num_WeightDEM_temp,Num_Query);
    for DEM_i=1:Num_WeightDEM_temp
        PostPDF_DEMTemp(DEM_i,:)=sum(Post_PDFWeight(ID_PDFTable(:,4)==DEM_i,:));
    end
    [PostPDF_DEMTemp,SumPDFDEM_Post]=PDF_NormFunc(PostPDF_DEMTemp,PriorPDF_DEM(:,2:end));
end
PostPDF_DEM(:,1)=PostPDF_DEMTemp;

% update the PDF_DPM
SumDPMPDF_Post=zeros(3,Num_Query);% 3*Num_Query
Num_WeightDPM=[size(PriorDPMPDF_Safety,1),size(PriorDPMPDF_Comfort,1),size(PriorDPMPDF_Efficiency,1)];

% Update the PDFDPM_Safety
PostPDFDPM_Safety=PriorDPMPDF_Safety;
PostPDF_DPMTemp=zeros(Num_WeightDPM(1),Num_Query);
for NumWeight_i=1:Num_WeightDPM(1)
    PostPDF_DPMTemp(NumWeight_i,:)=sum(Post_PDFWeight(ID_PDFTable(:,1)==NumWeight_i,:));
end
[PostDPMPDFWeight_Temp,SumPostPDFDPM_Temp]=PDF_NormFunc(PostPDF_DPMTemp,PriorDPMPDF_Safety(:,2:end));
PostPDFDPM_Safety(:,1)=PostDPMPDFWeight_Temp;
SumDPMPDF_Post(1,:)=SumPostPDFDPM_Temp;

% Update the PDFDPM_Comfort
PostPDFDPM_Comfort=PriorDPMPDF_Comfort;
PostPDF_DPMTemp=zeros(Num_WeightDPM(2),Num_Query);
for NumWeight_i=1:Num_WeightDPM(2)
    PostPDF_DPMTemp(NumWeight_i,:)=sum(Post_PDFWeight(ID_PDFTable(:,2)==NumWeight_i,:));
end
[PostDPMPDFWeight_Temp,SumPostPDFDPM_Temp]=PDF_NormFunc(PostPDF_DPMTemp,PriorDPMPDF_Comfort(:,2:end));
PostPDFDPM_Comfort(:,1)=PostDPMPDFWeight_Temp;
SumDPMPDF_Post(2,:)=SumPostPDFDPM_Temp;

% Update the PDFDPM_Efficiency
PostPDFDPM_Efficiency=PriorDPMPDF_Efficiency;
PostPDF_DPMTemp=zeros(Num_WeightDPM(3),Num_Query);
for NumWeight_i=1:Num_WeightDPM(3)
    PostPDF_DPMTemp(NumWeight_i,:)=sum(Post_PDFWeight(ID_PDFTable(:,3)==NumWeight_i,:));
end
[PostDPMPDFWeight_Temp,SumPostPDFDPM_Temp]=PDF_NormFunc(PostPDF_DPMTemp,PriorDPMPDF_Efficiency(:,2:end));
PostPDFDPM_Efficiency(:,1)=PostDPMPDFWeight_Temp;
SumDPMPDF_Post(3,:)=SumPostPDFDPM_Temp;
end

function [post_prob,sum_prob]=PDF_NormFunc(PDF,Weight_Set)
    % prob_distrib is a array of the post probability distribution. the row
    % number is the dicrete weight number,and the column number is the query/action.
    % each column is the post prob distribution of the query.
    % this function is to calculate the total prob in the considering
    % weight range to be 1
    % pdf_func: is a function handle.
   if size(PDF,1)==1
        post_prob=1;
        sum_prob=PDF;
    else
        uniqueweight=unique(Weight_Set(:,1));
        Interval_Weight=min(diff(uniqueweight));
        Ndim_ValidWeight=size(Weight_Set,2)-1;
        % considering the truth that the valid range of the independent variable
        if Ndim_ValidWeight==1
            sum_prob=sum(PDF(1:end-1))*Interval_Weight;
        else 
            pos_temp=sum(Weight_Set(:,1:Ndim_ValidWeight),2)<=1-Interval_Weight;
            sum_prob=sum(PDF(pos_temp,:))*Interval_Weight^Ndim_ValidWeight;
        end
        post_prob=PDF./repmat(sum_prob,size(PDF,1),1);
    end        
end

== matlab function Prescan_Carsim_0118_cs/BMW_X5_SUV_1/DEM updating and Preference Estimation/UpdateDEM/Trajectory Planning Parameter Management2/Determine planning parameter according to the expected TrajectoryIndicators_LookUpTable ==
  data: unused input; PlanningParameter output size=[9,1]; ExpectedNext_QueryID input; Parameter_IndicatorLookUpTable input
function PlanningParameter = fcn(~, ExpectedNext_QueryID,Parameter_IndicatorLookUpTable)

persistent Parameter_Indicator_LookUpTable
if isempty(Parameter_Indicator_LookUpTable)
    Parameter_Indicator_LookUpTable=Parameter_IndicatorLookUpTable;
end

PlanningParameter=Parameter_Indicator_LookUpTable(ExpectedNext_QueryID,1:9)';
end

== matlab function Prescan_Carsim_0118_cs/BMW_X5_SUV_1/DEM updating and Preference Estimation/UpdateDEM/Construct Comparison Group/Comparison Group_1 ==
  data: FeedBack output; Feedback_Driver input; Real_Trajectory_Indicator input size=[1 3]; TrajectoryIndicatorRange input; Query_Compare output size=[1 3]; NormalisedTrajectoryIndicator_Pool input; Evaluated_NormalisedTrajectoryIndicator output size=[21,1]; LastPreference_Normalised output
function [FeedBack,Query_Compare,Evaluated_NormalisedTrajectoryIndicator,LastPreference_Normalised] = fcn(Feedback_Driver,Real_Trajectory_Indicator,TrajectoryIndicatorRange,NormalisedTrajectoryIndicator_Pool)
% Construct the Query_Compare corresponding to the feedback

Real_NormalisedTrajectory_Indicator=DriverPerceptionModel(Real_Trajectory_Indicator,0,TrajectoryIndicatorRange);
Diff_TrajectoryInd=NormalisedTrajectoryIndicator_Pool-repmat(Real_NormalisedTrajectory_Indicator,size(NormalisedTrajectoryIndicator_Pool,1),1);
[~,Minimum_No]=min(sum(Diff_TrajectoryInd.^2,2));

%=========== Initialization
persistent LastPreference_TrajectoryIndicator LastPreference_NormalisedTrajectoryIndicator
if isempty(LastPreference_TrajectoryIndicator)
    LastPreference_TrajectoryIndicator=Real_Trajectory_Indicator;
    LastPreference_NormalisedTrajectoryIndicator=Real_NormalisedTrajectory_Indicator;
end

persistent Evaluated_NormalisedIndicator Step
if isempty(Evaluated_NormalisedIndicator)
    Step=1; 
    Evaluated_NormalisedIndicator=zeros(size(NormalisedTrajectoryIndicator_Pool,1),1);
    Evaluated_NormalisedIndicator(Step)=Minimum_No;
    Step=Step+1;
end

%==============
FeedBack=Feedback_Driver;
% Update the evaluated indicator
if not(ismember(Minimum_No,unique(Evaluated_NormalisedIndicator)))
    Evaluated_NormalisedIndicator(Step)=Minimum_No;      
    Step=Step+1;
end

Query_Compare=Real_NormalisedTrajectory_Indicator-LastPreference_NormalisedTrajectoryIndicator;
Evaluated_NormalisedTrajectoryIndicator=Evaluated_NormalisedIndicator;

if Feedback_Driver==2
    LastPreference_TrajectoryIndicator=Real_Trajectory_Indicator;
    LastPreference_NormalisedTrajectoryIndicator=Real_NormalisedTrajectory_Indicator;
end
LastPreference_Normalised=LastPreference_NormalisedTrajectoryIndicator;
end

% Local Functions================
function TrajectoryIndicator_Perceived=DriverPerceptionModel(TrajectoryIndicator,Flag,TrajectoryIndicatorRange)
% Flag: 0 means to transform the real trajectory indicator into Normalized
% Trajectory Indicators, vice versa, 1 means transform the normalized into
% real trajectory indicators

% RightLateralOffset,LateralAcceleration,Time
% Minimum_TrajectoryIndicator=[0,0.4,14];
% Maximum_TrajectoryIndicator=[0.5,3.4,18];
Minimum_TrajectoryIndicator=TrajectoryIndicatorRange(1,:);
Maximum_TrajectoryIndicator=TrajectoryIndicatorRange(2,:);

if Flag==1
    Normalized_TrajectoryIndicator=TrajectoryIndicator;
    TrajectoryIndicator_Perceived=Minimum_TrajectoryIndicator+(Maximum_TrajectoryIndicator-Minimum_TrajectoryIndicator).*Normalized_TrajectoryIndicator;
    % This is special for the LateralOffset_Right
    TrajectoryIndicator_Perceived(1)=-1*TrajectoryIndicator_Perceived(1);
elseif Flag==0
    %==== These are refered to the DriverPerceptionBase.m
    % JND-just noticeable difference
    %Can You Feel The Difference? The Just Noticeable Difference of
    %Longitudinal Acceleration, http://sage.cnpereading.com/paragraph/article/?doi=10.1177/1541931213571271
    JND_Acceleration=0.1;
    % Lateral Offset, Assume Left and Right be tha same,and to be 0.1m;
    JND_LateralOffset=0.1;%
    % Time, Or May be the Average Time would be More Significant
    JND_Time=2;
    
    GridIndicator=zeros(3,size(Minimum_TrajectoryIndicator,2));
    GridIndicator(1,:)=(Minimum_TrajectoryIndicator+eps)./[JND_LateralOffset,JND_Acceleration,JND_Time];
    GridIndicator(2,:)=(Maximum_TrajectoryIndicator+eps)./[JND_LateralOffset,JND_Acceleration,JND_Time];
    GridIndicator(3,:)=(abs(TrajectoryIndicator)+eps)./[JND_LateralOffset,JND_Acceleration,JND_Time];
    
    TrajectoryIndicator_Perceived=(GridIndicator(3,:)-GridIndicator(1,:))./(GridIndicator(2,:)-GridIndicator(1,:));
    TrajectoryIndicator_Perceived(TrajectoryIndicator_Perceived<0)=0;
    TrajectoryIndicator_Perceived(TrajectoryIndicator_Perceived>1)=1;
end
end

== matlab function Prescan_Carsim_0118_cs/BMW_X5_SUV_1/Tracking Control & vehicle dynamics/Lane Keeping Assistance/Path Tracking - LQR controller1/LQR Feedforward ==
  data: Feedforward output; PreviewDistance input; Curvature input; v input
function Feedforward = fcn(PreviewDistance, Curvature,v)
% LQR前馈量计算，与赵斌的SMC前馈量计算完全一致
%先定义车辆本身的参数
g=9.8;%重力加速度m/s^2
%{
%=============== Original Vehicle Parameters
M=1396; %车辆的质量kg
I=2204; %车辆的横摆转动惯量kg·m2
Kf=50192; %前轮的侧偏刚度Nm/rad
Kr=50192; %后轮的侧偏刚度Nm/rad
Lf=1.01; %车辆质心到前轴的距离m
Lr=1.59; %车辆质心到后轴的距离m
%}
%=====The JTEKT vehicle Parameter
M=1275; %车辆的质量kg
I=1523; %车辆的横摆转动惯量kg·m2
Kf=20000; %Calculated According to the carsim vehicle tire (under Fn=3500N)
Kr=20000; %后轮的侧偏刚度Nm/rad
Lf=1.016; %车辆质心到前轴的距离m
Lr=1.644; %车辆质心到后轴的距离m



%待调参数： 预瞄时长t_pre, 滑膜面参数 c1, c2, 趋近率参数delta, kapa
%输入参数； 预瞄偏差ep,  参考航向角phi_d, 本车航向角 phi, 道路曲率 qulv  航向角偏差影响系数 phir_k0 phir_k1
L = PreviewDistance; %车辆预瞄距离设定
smc_a34 = (Kf+Kr)/M+L*(Kf*Lf-Kr*Lr)/I;
smc_b32 = (L*Kf*Lf)/I+Kf/M;
k3 = smc_a34/smc_b32;
Feedforward= (M*v^2*Curvature)/(2*(Lf+Lr))*(Lr/Kf-Lf/Kr+Lf/Kr*k3)+Curvature*((Lf+Lr)-Lr*k3);
